simulink model "after_tick_eg_2018a"  (R2018a)
settings: Solver=VariableStepAuto  StartTime=0.0  StopTime=10.0  RelTol=1e-3
settings Model: Creator=86188  LastModifiedBy=86188

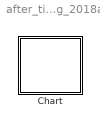
== system after_tick_eg_2018a ==
  Chart : Stateflow chart  TreatAsAtomicUnit=on

== stateflow chart after_tick_eg_2018a/Chart ==
  state A
    en:f("en_A");
    du:f("du_A");
  state B
    en:f("en_B")
    du:f("du_B");
  (default) -> A
  A -> B : after(10,tick)
  B -> A : after(10,tick)
  data: s function_input
  function f(s):
    | function f(s)
    |   fprintf(s+"\n");
